simulink model "my_dom_trans"  (R2018a)
settings: Solver=VariableStepAuto  StartTime=0.0  StopTime=10000  RelTol=1e-3
values from neighbouring files (symbols this model uses):
  d_T_z = 0    [leveled_NL.m]    (also in leveled_transmitancja.m)
  d_T_zew = 0    [leveled_NL.m]    (also in leveled_transmitancja.m = 2)
  steptime = 1000    [leveled_NL.m]    (also in leveled_transmitancja.m)
  T_p0 = (K_1*T_wew0+K_p*T_zew1)*M    [leveled_NL.m]    (also in leveled_transmitancja.m)
  T_wew0 = (c_p*ro_p*f_p1*T_z1+K_1*K_p*T_zew1*M +K_w*T_zew1)/(c_p*ro_p*f_p1+K_1+K_w-(K_1^2)*M)    [leveled_NL.m]    (also in leveled_transmitancja.m)
undefined symbols (not defined in the file or in its folder): L1, L2, M1, M2
settings Model: Creator=johnb  LastModifiedBy=johnb

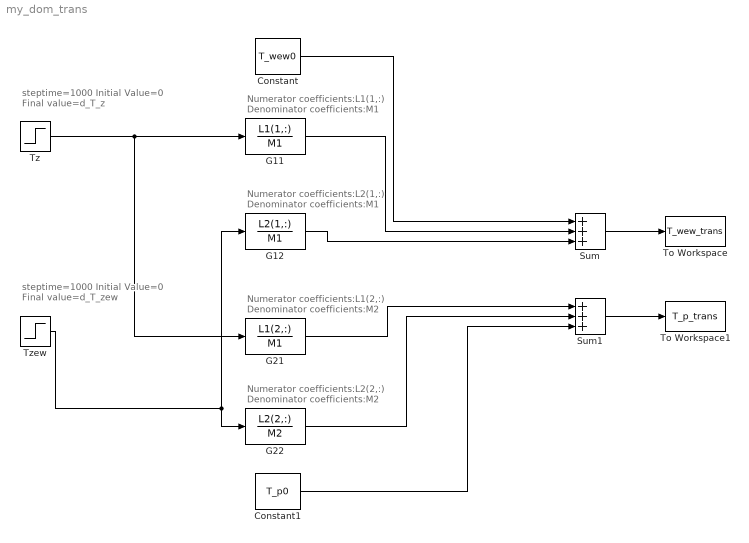
== system my_dom_trans ==
  note: Numerator coefficients:L1(1,:)
      | Denominator coefficients:M1
  note: steptime=1000
      | Initial Value=0
      | Final value=d_T_z
  note: steptime=1000
      | Initial Value=0
      | Final value=d_T_zew
  note: Numerator coefficients:L2(1,:)
      | Denominator coefficients:M1
  note: Numerator coefficients:L1(2,:)
      | Denominator coefficients:M2
  note: Numerator coefficients:L2(2,:)
      | Denominator coefficients:M2
  Constant : Constant  Value=T_wew0
  Constant1 : Constant  Value=T_p0
  G11 : TransferFcn  Numerator=L1(1,:)  Denominator=M1
  G12 : TransferFcn  Numerator=L2(1,:)  Denominator=M1
  G21 : TransferFcn  Numerator=L1(2,:)  Denominator=M1
  G22 : TransferFcn  Numerator=L2(2,:)  Denominator=M2
  Sum : Sum  Inputs=3
  Sum1 : Sum  Inputs=3
  To Workspace : ToWorkspace  VariableName=T_wew_trans  SaveFormat=Timeseries  SampleTime=-1
  To Workspace1 : ToWorkspace  VariableName=T_p_trans  SaveFormat=Timeseries  SampleTime=-1
  Tz : Step  Time=steptime  After=d_T_z  SampleTime=0
  "Tzew " : Step  Time=steptime  After=d_T_zew  SampleTime=0
  wires:
  Sum/1 -> To Workspace/1
  Sum1/1 -> To Workspace1/1
  Tz/1 -> G11/1, G21/1
  "Tzew "/1 -> G12/1, G22/1
  Constant/1 -> Sum/1
  G11/1 -> Sum/2
  G12/1 -> Sum/3
  G21/1 -> Sum1/1
  G22/1 -> Sum1/2
  Constant1/1 -> Sum1/3
